simulink model "sim_with_disturbances"  (R2025b)
settings: Solver=VariableStepAuto  StartTime=0.0  StopTime=Tend  RelTol=1e-3
undefined symbols (not defined in the file): delta_1, delta_2, rho, Ts
libraries: cstblocks x2, simulink x2
settings Model: Creator=davidecovolo  LastModifiedBy=davidecovolo

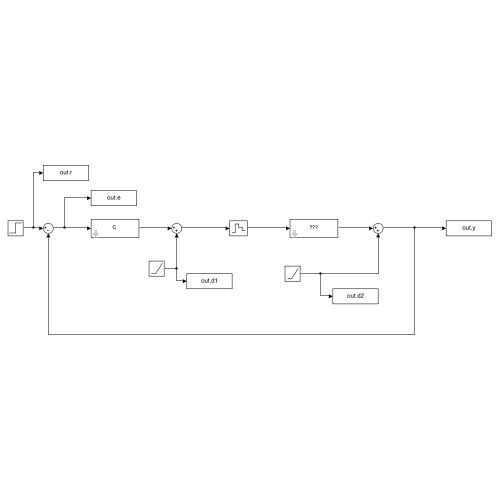
[thumbnail: Simulink's stored preview of the top-level diagram]
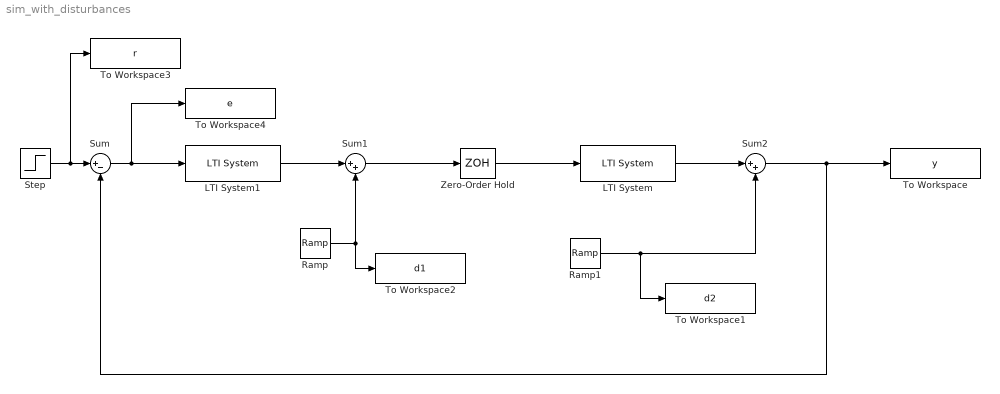
== system sim_with_disturbances ==
  LTI System : cstblocks/LTI System  sys=G_ct  IC=[]  PadeOrder=0
  LTI System1 : cstblocks/LTI System  sys=C  IC=[]  PadeOrder=0
  Ramp : simulink/Sources/Ramp  slope=delta_1  start=0  InitialOutput=0
  Ramp1 : simulink/Sources/Ramp  slope=delta_2  start=0  InitialOutput=0
  Step : Step  Time=0  After=rho  SampleTime=0
  Sum : Sum  Inputs=|+-
  Sum1 : Sum  Inputs=|++
  Sum2 : Sum  Inputs=|++
  To Workspace : ToWorkspace  VariableName=y  SaveFormat=Timeseries  SampleTime=Ts*0.001
  To Workspace1 : ToWorkspace  VariableName=d2  SaveFormat=Timeseries  SampleTime=Ts*0.001
  To Workspace2 : ToWorkspace  VariableName=d1  SaveFormat=Timeseries  SampleTime=Ts*0.001
  To Workspace3 : ToWorkspace  VariableName=r  SaveFormat=Timeseries  SampleTime=Ts*0.001
  To Workspace4 : ToWorkspace  VariableName=e  SaveFormat=Timeseries  SampleTime=Ts*0.001
  Zero-Order Hold : ZeroOrderHold  SampleTime=Ts
  wires:
  LTI System1/1 -> Sum1/1
  Sum1/1 -> Zero-Order Hold/1
  Zero-Order Hold/1 -> LTI System/1
  LTI System/1 -> Sum2/1
  Ramp1/1 -> To Workspace1/1, Sum2/2
  Ramp/1 -> Sum1/2, To Workspace2/1
  Sum2/1 -> Sum/2, To Workspace/1
  Step/1 -> To Workspace3/1, Sum/1
  Sum/1 -> To Workspace4/1, LTI System1/1
